simulink model "takeoffANDlandingV5_23b"  (R2023b)
settings: Solver=ode4  StartTime=0.0  StopTime=450  FixedStep=0.001  RelTol=1e-3
values from neighbouring files (symbols this model uses):
  a0 = 340.294    [basedata.m]    (also in basedata.mat; control_design.mat; landing_init.m; landing_plan.mat)
  b_ref = 2.0    (= 2)    [basedata.m]    (also in basedata.mat; control_design.mat; landing_init.m; landing_plan.mat)
  c_gear = [0.8e4, 1.4e4, 1.4e4]    [basedata.m]    (also in basedata.mat = [8000 14000 14000]; control_design.mat = [8000 14000 14000]; landing_init.m; landing_plan.mat = [8000 14000 14000])
  c_lat = [1.4e4, 2.2e4, 2.2e4]    [basedata.m]    (also in basedata.mat = [14000 22000 22000]; control_design.mat = [14000 22000 22000]; landing_init.m; landing_plan.mat = [14000 22000 22000])
  c_ref = 0.9    [basedata.m]    (also in basedata.mat; control_design.mat; landing_init.m; landing_plan.mat)
  c_roll = [0.020, 0.018, 0.018]    [basedata.m]    (also in basedata.mat = [0.02 0.018 0.018]; control_design.mat = [0.02 0.018 0.018]; landing_init.m; landing_plan.mat = [0.02 0.018 0.018])
  CD0 = 0.045    [basedata.m]    (also in basedata.mat; canshujisuan.m; control_design.mat; landing_init.m)
  CL0 = 0.083    [basedata.m]    (also in basedata.mat; control_design.mat; landing_init.m; landing_plan.mat)
  CLa = 3.80    (= 3.8)    [basedata.m]    (also in basedata.mat; canshujisuan.m = 2.5; control_design.mat; landing_init.m)
  Clb = -0.08    [basedata.m]    (also in basedata.mat; control_design.mat; landing_init.m; landing_plan.mat)
  Clda = -0.20    (= -0.2)    [basedata.m]    (also in basedata.mat; control_design.mat; landing_init.m; landing_plan.mat)
  CLde = 0.28    [basedata.m]    (also in basedata.mat; control_design.mat; landing_init.m; landing_plan.mat)
  Clp = -0.70    (= -0.7)    [basedata.m]    (also in basedata.mat; control_design.mat; landing_init.m; landing_plan.mat)
  CLq = 4.50    (= 4.5)    [basedata.m]    (also in basedata.mat; canshujisuan.m = 3; control_design.mat; landing_init.m)
  Clr = 0.08    [basedata.m]    (also in basedata.mat; control_design.mat; landing_init.m; landing_plan.mat)
  Cm0 = 0.060    (= 0.06)    [basedata.m]    (also in basedata.mat; control_design.mat; landing_init.m; landing_plan.mat)
  Cma = -0.80    (= -0.8)    [basedata.m]    (also in basedata.mat; control_design.mat; landing_init.m; landing_plan.mat)
  Cmde = -0.90    (= -0.9)    [basedata.m]    (also in basedata.mat; control_design.mat; landing_init.m; landing_plan.mat)
  Cmq = -18.0    (= -18)    [basedata.m]    (also in basedata.mat; control_design.mat; landing_init.m; landing_plan.mat)
  Cnb = 0.25    [basedata.m]    (also in basedata.mat; control_design.mat; landing_init.m; landing_plan.mat)
  Cndr = -0.15    [basedata.m]    (also in basedata.mat; control_design.mat; landing_init.m; landing_plan.mat)
  Cnp = -0.04    [basedata.m]    (also in basedata.mat; control_design.mat; landing_init.m; landing_plan.mat)
  Cnr = -0.45    [basedata.m]    (also in basedata.mat; control_design.mat; landing_init.m; landing_plan.mat)
  CSb = -0.70    (= -0.7)    [basedata.m]    (also in basedata.mat; control_design.mat; landing_init.m; landing_plan.mat)
  CSdr = 0.18    [basedata.m]    (also in basedata.mat; control_design.mat; landing_init.m; landing_plan.mat)
  CSr = 0.12    [basedata.m]    (also in basedata.mat; control_design.mat; landing_init.m; landing_plan.mat)
  D = 0.5 * rho0 * V^2 * S_ref * CD_current    [canshujisuan.m]
  D0 = 1400    [basedata.m]    (also in basedata.mat; control_design.mat = 800; landing.m; landing_init.m)
  da_max = 25    [basedata.m]    (also in basedata.mat; control_design.mat; landing_init.m; landing_plan.mat)
  da_min = -da_max    (= -25)    [basedata.m]    (also in basedata.mat; control_design.mat; landing_init.m; landing_plan.mat)
  de_max = 25    [basedata.m]    (also in basedata.mat; control_design.mat; landing_init.m; landing_plan.mat)
  de_min = -de_max    (= -25)    [basedata.m]    (also in basedata.mat; control_design.mat; landing_init.m; landing_plan.mat)
  DH = pi / 180    (= 0.0174532925199)    [basedata.m]    (also in basedata.mat; control_design.mat; landing_init.m; landing_plan.mat)
  dr_max = 25    [basedata.m]    (also in basedata.mat; control_design.mat; landing_init.m; landing_plan.mat)
  dr_min = -dr_max    (= -25)    [basedata.m]    (also in basedata.mat; control_design.mat; landing_init.m; landing_plan.mat)
  g = 9.80665    [basedata.m]    (also in basedata.mat; canshujisuan.m; control_design.mat; landing_init.m)
  ground_z = 0.0    (= 0)    [basedata.m]    (also in basedata.mat; control_design.mat; landing_init.m; landing_plan.mat)
  H_B = 132.622761894    [basedata.mat]    (also in landing_trajectory.m = H_R - R * cos(a1); landingplan.mat)
  H_C = 72.1000994005    [basedata.mat]    (also in landing_trajectory.m = H_R - R * cos(a2); landingplan.mat)
  H_climb_complete = 1000    [control_design.mat]    (also in landing.m; landing_init.m; landing_plan.mat; landingplan.mat)
  H_entry = 1000    [basedata.mat]    (also in landing_trajectory.m; landingplan.mat)
  H_exp = 20    [basedata.mat]    (also in landing_trajectory.m; landingplan.mat)
  HD = 180 / pi    (= 57.2957795131)    [basedata.m]    (also in basedata.mat; control_design.mat; landing_init.m; landing_plan.mat)
  I = [ Ixx, -Ixy, -Ixz ... (first row only)    [basedata.m]    (also in basedata.mat = [120  0  0; 0  480  0; 0  0  520]; control_design.mat = [120  0  0; 0  480  0; 0  0  520]; landing_init.m; landing_plan.mat = [120  0  0; 0  480  0; 0  0  520])
  K = 0.12    [basedata.m]    (also in basedata.mat; canshujisuan.m = 0.08; control_design.mat; landing_init.m)
  K_alpha = 7.5375    [basedata.mat]    (also in control_design.m = (((wd_pitch^2)-a24))/(2*kesi_pitch*wd_pitch); control_design.mat; controller.m = 5; landingplan.mat)
  k_gear = [1.0e5, 3.0e5, 3.0e5]    [basedata.m]    (also in basedata.mat = [100000 300000 300000]; control_design.mat = [100000 300000 300000]; landing_init.m; landing_plan.mat = [100000 300000 300000])
  Kn_pitch = -0.120095403309    [basedata.mat]    (also in control_design.m = -(2.2*g*(wd_pitch)^2)/(Tr*(((wd_pitch)^2)-a24)*V_control*a34; control_design.mat; controller.m = (2.2*wd^2*g)/(Tr*(wd^2-a24)*V_test*a34); landingplan.mat)
  Kw_pitch = -0.483749055178    [basedata.mat]    (also in control_design.m = -2*kesi_pitch*wd_pitch/a25; control_design.mat; controller.m = -(2*zeta*wd) / a25; landingplan.mat)
  m = 600.0    (= 600)    [basedata.m]    (also in basedata.mat; canshujisuan.m; control_design.mat; landing_init.m)
  mu_brake = [0.0, 0.55, 0.55]    [basedata.m]    (also in basedata.mat = [0 0.55 0.55]; control_design.mat = [0 0.55 0.55]; landing_init.m; landing_plan.mat = [0 0.55 0.55])
  phi0 = 0    [control_design.mat]    (also in landing.m; landing_init.m; landing_init.mat; landing_plan.mat)
  psi0 = 0    [control_design.mat]    (also in landing.m; landing_init.m; landing_init.mat; landing_plan.mat)
  r_left_b = r_gear_b(:,2)    [basedata.m]    (also in basedata.mat = [-0.333333333333 -0.8 0.65]; control_design.mat = [-0.333333333333 -0.8 0.65]; landing_init.m; landing_plan.mat = [-0.333333333333 -0.8 0.65])
  r_nose_b = r_gear_b(:,1)    [basedata.m]    (also in basedata.mat = [2 0 0.65]; control_design.mat = [2 0 0.65]; landing_init.m; landing_plan.mat = [2 0 0.65])
  r_right_b = r_gear_b(:,3)    [basedata.m]    (also in basedata.mat = [-0.333333333333 0.8 0.65]; control_design.mat = [-0.333333333333 0.8 0.65]; landing_init.m; landing_plan.mat = [-0.333333333333 0.8 0.65])
  rho0 = 1.225    [basedata.m]    (also in basedata.mat; canshujisuan.m; control_design.mat; landing_init.m)
  S_ref = 1.2    [basedata.m]    (also in basedata.mat; canshujisuan.m; control_design.mat; landing_init.m)
  theta0 = 0    [control_design.mat]    (also in landing.m; landing_init.m; landing_init.mat = 0.0523598775598; landing_plan.mat = 0.0523560209424)
  u0_b = 0    [control_design.mat]    (also in landing.m = 128; landing_init.m = 128; landing_init.mat = 100; landing_plan.mat = 128)
  v0_b = 0    [control_design.mat]    (also in landing.m; landing_init.m; landing_init.mat; landing_plan.mat)
  V_app = 128.516392565    [basedata.mat]    (also in landing_trajectory.m = 1.4 * Vs; landingplan.mat)
  V_cruise = 200    [basedata.m]
  v_eps = 0.20    (= 0.2)    [basedata.m]    (also in basedata.mat; control_design.mat; landing_init.m; landing_plan.mat)
  V_flare = V_shallow    [landing_trajectory.m]
  V_min = 3    [control_design.mat]    (also in landing.m; landing_init.m; landing_plan.mat; landingplan.mat)
  V_shallow = 110.156907913    [basedata.mat]    (also in landing_trajectory.m = 1.2 * Vs; landingplan.mat)
  w0_b = 0    [control_design.mat]    (also in landing.m; landing_init.m; landing_init.mat; landing_plan.mat)
  wheel_radius = 0.18    [basedata.m]    (also in basedata.mat; control_design.mat; landing_init.m; landing_plan.mat)
  WOW_on = 0.000    (= 0)    [basedata.m]    (also in basedata.mat; control_design.mat; landing_init.m; landing_plan.mat)
  Xg0 = 0    [control_design.mat]    (also in landing.m = -12000; landing_init.m = -12000; landing_init.mat = -8000; landing_plan.mat = -12000)
  Yg0 = 3    [control_design.mat]    (also in landing.m = 0; landing_init.m = 0; landing_init.mat = 0; landing_plan.mat = 0)
  Zg0 = ground_z - wheel_radius - r_gear_b(3,1) + static_deflection    [basedata.m]    (also in basedata.mat = -0.8215943; control_design.mat = -0.8215943; landing.m = -1000; landing_init.m = -1000)
undefined symbols (not defined in the file or in its folder): H_start, I_xz, I_yz, Ix_Iy, Iy_Iz, Iz_Ix, X_landing_start
libraries: simulink x54, matrix_library x19
(part 1 of 4)
settings Model: SimulationMode=accelerator  Creator=34355  LastModifiedBy=34355
settings RTWCC: GPUComputeCapability=5.0

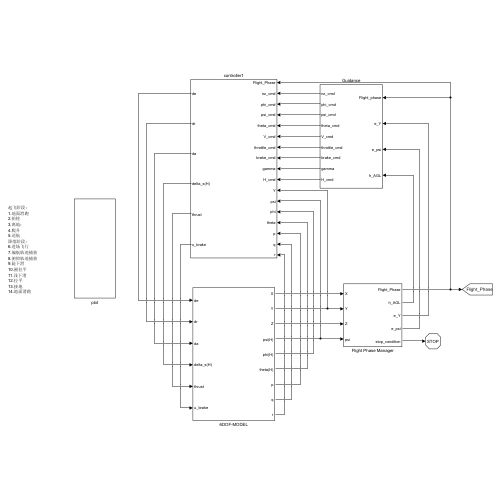
[thumbnail: Simulink's stored preview of the top-level diagram]
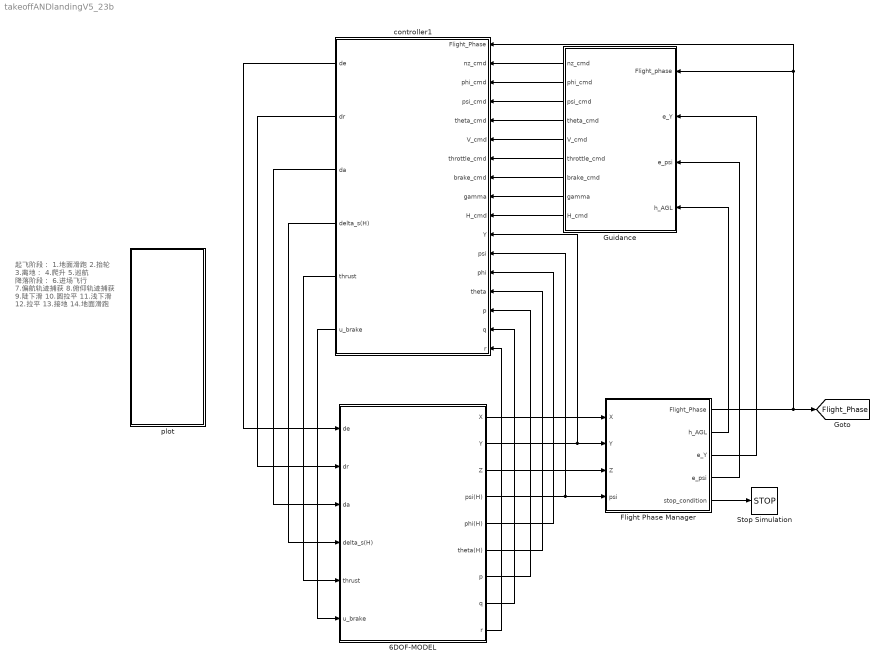
== system takeoffANDlandingV5_23b ==
  note: 起飞阶段：
      | 1.地面滑跑
      | 2.抬轮
      | 3.离地：
      | 4.爬升
      | 5.巡航
      | 降落阶段：
      | 6.进场飞行
      | 7.偏航轨迹捕获
      | 8.俯仰轨迹捕获
      | 9.陡下滑
      | 10.圆拉平
      | 11.浅下滑
      | 12.拉平
      | 13.接地
      | 14.地面滑跑
  6DOF-MODEL : Subsystem
  Flight Phase Manager : Subsystem
  Guidance : Subsystem
  Stop Simulation : Stop
  controller1 : Subsystem
  plot : Subsystem
  tag scope: Flight_Phase=global
  wires:
  controller1/1(de) -> 6DOF-MODEL/1(de)
  controller1/2(dr) -> 6DOF-MODEL/2(dr)
  controller1/3(da) -> 6DOF-MODEL/3(da)
  controller1/4(delta_s(H)) -> 6DOF-MODEL/4(delta_s(H))
  controller1/5(thrust) -> 6DOF-MODEL/5(thrust)
  controller1/6(u_brake) -> 6DOF-MODEL/6(u_brake)
  Flight Phase Manager/1(Flight_Phase) -> [Flight_Phase], Guidance/1(Flight_phase), controller1/1(Flight_Phase)
  Flight Phase Manager/3(e_Y) -> Guidance/2(e_Y)
  Flight Phase Manager/4(e_psi) -> Guidance/3(e_psi)
  Flight Phase Manager/2(h_AGL) -> Guidance/4(h_AGL)
  Guidance/1(nz_cmd) -> controller1/2(nz_cmd)
  Guidance/2(phi_cmd) -> controller1/3(phi_cmd)
  Guidance/4(theta_cmd) -> controller1/5(theta_cmd)
  Guidance/5(V_cmd) -> controller1/6(V_cmd)
  Guidance/6(throttle_cmd) -> controller1/7(throttle_cmd)
  Guidance/7(brake_cmd) -> controller1/8(brake_cmd)
  Guidance/8(gamma) -> controller1/9(gamma)
  Guidance/9(H_cmd) -> controller1/10(H_cmd)
  Flight Phase Manager/5(stop_condition) -> Stop Simulation/1
  Guidance/3(psi_cmd) -> controller1/4(psi_cmd)
  6DOF-MODEL/1(X) -> Flight Phase Manager/1(X)
  6DOF-MODEL/2(Y) -> controller1/11(Y), Flight Phase Manager/2(Y)
  6DOF-MODEL/3(Z) -> Flight Phase Manager/3(Z)
  6DOF-MODEL/4(psi(H)) -> Flight Phase Manager/4(psi), controller1/12(psi)
  6DOF-MODEL/5(phi(H)) -> controller1/13(phi)
  6DOF-MODEL/6(theta(H)) -> controller1/14(theta)
  6DOF-MODEL/7(p) -> controller1/15(p)
  6DOF-MODEL/8(q) -> controller1/16(q)
  6DOF-MODEL/9(r) -> controller1/17(r)

== system takeoffANDlandingV5_23b/6DOF-MODEL ==
  de : Inport
  dr : Inport  Port=2
  da : Inport  Port=3
  delta_s(H) : Inport  Port=4
  thrust : Inport  Port=5
  u_brake : Inport  Port=6
  AERO-PARAMETER : Subsystem
  Scope : Scope
  Scope5 : Scope
  Scope6 : Scope
  动力学 : Subsystem
  X : Outport
  Y : Outport  Port=2
  Z : Outport  Port=3
  psi(H) : Outport  Port=4
  phi(H) : Outport  Port=5
  theta(H) : Outport  Port=6
  p : Outport  Port=7
  q : Outport  Port=8
  r : Outport  Port=9
  wires:
  动力学/1(alpha(D)) -> Scope/1, AERO-PARAMETER/1(alpha(D))
  thrust/1 -> 动力学/7(thrust)
  u_brake/1 -> 动力学/9(u_brake)
  AERO-PARAMETER/1(D) -> Scope6/1, 动力学/1(D)
  AERO-PARAMETER/2(L) -> Scope5/1, 动力学/2(L)
  AERO-PARAMETER/3(S) -> 动力学/3(S)
  AERO-PARAMETER/4(MX) -> 动力学/4(MX)
  AERO-PARAMETER/5(MY) -> 动力学/5(MY)
  AERO-PARAMETER/6(MZ) -> 动力学/6(MZ)
  delta_s(H)/1 -> 动力学/8(delta_s(H))
  动力学/2(beta(D)) -> AERO-PARAMETER/2(beta(D))
  动力学/3(p) -> p/1, AERO-PARAMETER/3(p(H))
  动力学/4(q) -> q/1, AERO-PARAMETER/4(q(H))
  动力学/5(r) -> r/1, AERO-PARAMETER/5(r(H))
  de/1 -> AERO-PARAMETER/6(de(D))
  dr/1 -> AERO-PARAMETER/7(dr(D))
  da/1 -> AERO-PARAMETER/8(da)
  动力学/7(Y) -> Y/1
  动力学/8(Z) -> Z/1
  动力学/11(psi(H)) -> psi(H)/1
  动力学/10(theta(H)) -> theta(H)/1
  动力学/6(X) -> X/1
  动力学/9(phi(H)) -> phi(H)/1

== system takeoffANDlandingV5_23b/Flight Phase Manager ==
  X : Inport
  Y : Inport  Port=2
  Z : Inport  Port=3
  psi : Inport  Port=4
  Data Pre-processing : Subsystem
  Phase Logic : Stateflow chart  TreatAsAtomicUnit=on
  Flight_Phase : Outport
  h_AGL : Outport  Port=2
  e_Y : Outport  Port=3
  e_psi : Outport  Port=4
  stop_condition : Outport  Port=5
  wires:
  X/1 -> Data Pre-processing/1(X)
  Y/1 -> Data Pre-processing/2(Y)
  Z/1 -> Data Pre-processing/3(Z)
  psi/1 -> Data Pre-processing/4(psi)
  Phase Logic/1(Flight_Phase) -> Flight_Phase/1
  Data Pre-processing/1(reach_VR) -> Phase Logic/1(reach_VR)
  Data Pre-processing/2(airborne) -> Phase Logic/2(airborne)
  Data Pre-processing/3(safe_climb) -> Phase Logic/3(safe_climb)
  Data Pre-processing/4(in_cruise) -> Phase Logic/4(in_cruise)
  Data Pre-processing/5(task_mode) -> Phase Logic/5(Task_Mode)
  Data Pre-processing/6(yaw_captrue) -> Phase Logic/6(yawcapture)
  Data Pre-processing/8(in_steep) -> Phase Logic/8(in_steep)
  Data Pre-processing/9(In_round) -> Phase Logic/9(in_round)
  Data Pre-processing/10(Slight decline) -> Phase Logic/10(Slight_decline)
  Data Pre-processing/11(in_flare) -> Phase Logic/11(in_Flare)
  Data Pre-processing/12(touch_ground) -> Phase Logic/12(touch_ground)
  Data Pre-processing/13(in_ground) -> Phase Logic/13(in_ground)
  Data Pre-processing/14(h_ALG) -> h_AGL/1
  Data Pre-processing/16(e_Y) -> e_Y/1
  Data Pre-processing/15(e_psi) -> e_psi/1
  Data Pre-processing/17(stop_condition) -> stop_condition/1
  Data Pre-processing/7(pitchcaptrue) -> Phase Logic/7(pitchcaptrue)

== system takeoffANDlandingV5_23b/Guidance ==
  Flight_phase : Inport
  e_Y : Inport  Port=2
  e_psi : Inport  Port=3
  h_AGL : Inport  Port=4
  Bus Selector : BusSelector  OutputSignals=nz_cmd,phi_cmd,psi_cmd,theta_cmd,V_cmd,throttle_cmd,brake_cmd,H_cmd,gamma
  Compare To Constant : simulink/Logic and Bit Operations/Compare To Constant  relop=<=  const=5  OutDataTypeStr=boolean
  Compare To Constant1 : simulink/Logic and Bit Operations/Compare To Constant  relop=>  const=5  OutDataTypeStr=boolean
  Gain : Gain  Gain=HD
  Gain1 : Gain  Gain=HD
  Merge : Merge
  Rate Limiter : RateLimiter  RisingSlewLimit=1*DH  FallingSlewLimit=-1*DH  SampleTimeMode=inherited
  Rate Limiter1 : RateLimiter  RisingSlewLimit=10*DH  FallingSlewLimit=-10*DH  SampleTimeMode=inherited
  Rate Limiter2 : RateLimiter  RisingSlewLimit=10*DH  FallingSlewLimit=-10*DH  SampleTimeMode=inherited
  Rate Limiter3 : RateLimiter  RisingSlewLimit=0.8  FallingSlewLimit=-0.8  SampleTimeMode=inherited
  Saturation : Saturate  UpperLimit=2  LowerLimit=-2
  Saturation2 : Saturate  UpperLimit=1  LowerLimit=0
  Saturation3 : Saturate  UpperLimit=1  LowerLimit=0
  Saturation4 : Saturate  UpperLimit=250  LowerLimit=0
  Scope : Scope
  Scope8 : Scope
  Scope9 : Scope
  起飞阶段 : Subsystem
  降落阶段 : Subsystem
  nz_cmd : Outport
  phi_cmd : Outport  Port=2
  psi_cmd : Outport  Port=3
  theta_cmd : Outport  Port=4
  V_cmd : Outport  Port=5
  throttle_cmd : Outport  Port=6
  brake_cmd : Outport  Port=7
  gamma : Outport  Port=8
  H_cmd : Outport  Port=9
  wires:
  Bus Selector/5 -> Saturation4/1  "<V_cmd>"
  Bus Selector/4 -> Rate Limiter/1  "<theta_cmd>"
  Saturation4/1 -> V_cmd/1
  Bus Selector/7 -> Saturation3/1  "<brake_cmd>"
  Rate Limiter2/1 -> psi_cmd/1
  Saturation/1 -> Rate Limiter3/1
  Saturation3/1 -> brake_cmd/1
  Saturation2/1 -> throttle_cmd/1
  Merge/1 -> Bus Selector/1
  [vzg] -> 起飞阶段/8(vzg), 降落阶段/6(vzg)
  Rate Limiter/1 -> theta_cmd/1, Gain1/1
  Bus Selector/2 -> Rate Limiter1/1  "<phi_cmd>"
  Bus Selector/8 -> H_cmd/1, Scope9/1  "<H_cmd>"
  [theta_eular] -> 降落阶段/8(theta_eular), 起飞阶段/10(theta_eular)
  降落阶段/1(Cmd_Bus) -> Merge/2
  Bus Selector/1 -> Saturation/1  "<nz_cmd>"
  h_AGL/1 -> 起飞阶段/7(h_ALG), 降落阶段/2(h_AGL)
  [vxg] -> 降落阶段/9(Vg)
  [phi_eular] -> 起飞阶段/9(phi_eular), 降落阶段/7(phi_eular)
  起飞阶段/1(Cmd_Bus) -> Merge/1
  Flight_phase/1 -> Compare To Constant/1, 起飞阶段/1(Flight_phase), 降落阶段/1(Flight_phase), Compare To Constant1/1
  Compare To Constant/1 -> 起飞阶段/Enable
  [r] -> 起飞阶段/4(r)
  [Vwind_ground] -> 起飞阶段/5(Vwind_ground), 降落阶段/3(Vwind_ground)
  e_psi/1 -> 起飞阶段/3(e_psi)
  Gain/1 -> Scope8/1
  e_Y/1 -> 起飞阶段/2(e_Y)
  Bus Selector/9 -> gamma/1, Gain/1  "<gamma>"
  Compare To Constant1/1 -> 降落阶段/Enable
  [Va_safe] -> 起飞阶段/6(Va_safe), 降落阶段/4(Va_safe)
  Rate Limiter3/1 -> nz_cmd/1
  Bus Selector/6 -> Saturation2/1  "<throttle_cmd>"
  Rate Limiter1/1 -> phi_cmd/1
  [X_positon] -> 降落阶段/5(x_pos)
  Bus Selector/3 -> Rate Limiter2/1  "<psi_cmd>"
  Gain1/1 -> Scope/1

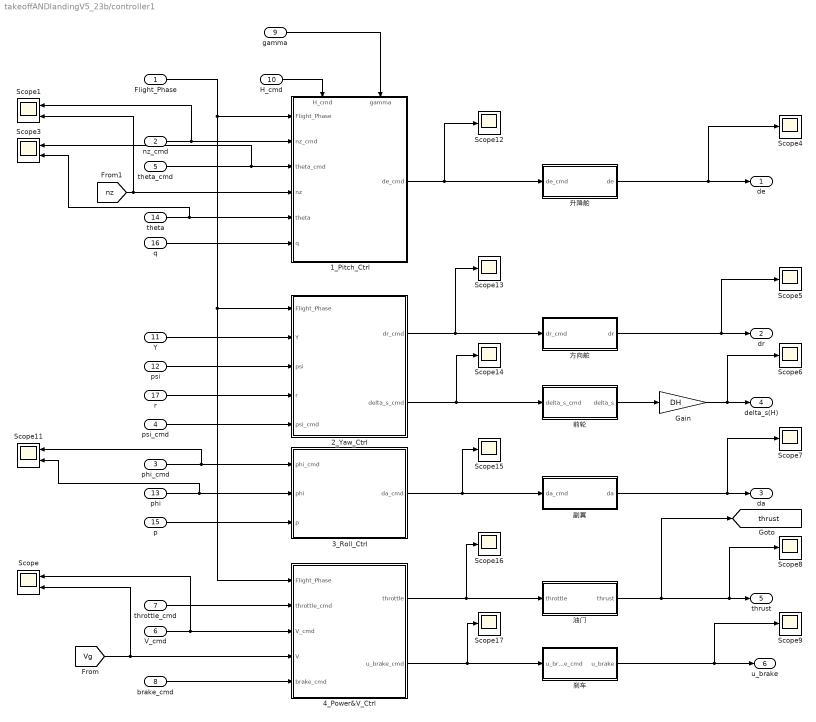
== system takeoffANDlandingV5_23b/controller1 ==
  Flight_Phase : Inport
  nz_cmd : Inport  Port=2
  phi_cmd : Inport  Port=3
  psi_cmd : Inport  Port=4
  theta_cmd : Inport  Port=5
  V_cmd : Inport  Port=6
  throttle_cmd : Inport  Port=7
  brake_cmd : Inport  Port=8
  gamma : Inport  Port=9
  H_cmd : Inport  Port=10
  Y : Inport  Port=11
  psi : Inport  Port=12
  phi : Inport  Port=13
  theta : Inport  Port=14
  p : Inport  Port=15
  q : Inport  Port=16
  r : Inport  Port=17
  1_Pitch_Ctrl : Subsystem
      settings: PortSchema="{\"entries\":[{\"content\":{\"sides\":[{\"content\":{\"connectorIds\":[\"In1\",\"In2\",\"In3\",\"In4\",\"In5\",\"In6\"]},\"type\":\"ConnectorPlacement.EquallySpacedRectSide\",\"uuid\":\"27d13232-9f89-4ac1-9c77-5758657de7c7\"},{\"content\":{\"connectorIds\":[\"Out1\"],\"side\":\"RIGHT\"},\"type\":\"ConnectorPlacement.EquallySpacedRectSide\",\"uuid\":\"ae62ad8c-a405-4422-b5ec-9ac723f70591\"},{\"content\":{\"connectorIds\":[\"In7\",\"In8\"],\"side\":\"TOP\"},\"type\":\"ConnectorPlacement.EquallySpacedRectSide\",\"uuid\":\"4cebe0f4-d768-4fb6-931c-2fd4183255b7\"}]},\"type\":\"ConnectorPlacement.EquallySpacedConnector\",\"uuid\":\"2c44e0df-7f94-4dab-9232-216c905b911f\"}],\"packageUris\":[\"http://schema.mathworks.com/mf0/Connector/R2020b\"],\"version\":\"1.0\"}"
  2_Yaw_Ctrl : Subsystem
  3_Roll_Ctrl : Subsystem
  4_Power&V_Ctrl : Subsystem
  Gain : Gain  Gain=DH
  Scope{,1,3,11} (4 alike) : Scope  NumInputPorts=2
  Scope{4..9,12..17} (12 alike) : Scope
  刹车 : Subsystem
  前轮 : Subsystem
  副翼 : Subsystem
  升降舵 : Subsystem
  方向舵 : Subsystem
  油门 : Subsystem
  de : Outport
  dr : Outport  Port=2
  da : Outport  Port=3
  delta_s(H) : Outport  Port=4
  thrust : Outport  Port=5
  u_brake : Outport  Port=6
  tag scope: thrust=global
  wires:
  phi_cmd/1 -> Scope11/1, 3_Roll_Ctrl/1(phi_cmd)
  phi/1 -> Scope11/2, 3_Roll_Ctrl/2(phi)
  p/1 -> 3_Roll_Ctrl/3(p)
  brake_cmd/1 -> 4_Power&V_Ctrl/5(brake_cmd)
  4_Power&V_Ctrl/1(throttle) -> 油门/1(throttle), Scope16/1
  Flight_Phase/1 -> 1_Pitch_Ctrl/1(Flight_Phase), 4_Power&V_Ctrl/1(Flight_Phase), 2_Yaw_Ctrl/1(Flight_Phase)
  nz_cmd/1 -> Scope1/1, 1_Pitch_Ctrl/2(nz_cmd)
  [nz] -> Scope1/2, 1_Pitch_Ctrl/4(nz)
  q/1 -> 1_Pitch_Ctrl/6(q)
  V_cmd/1 -> 4_Power&V_Ctrl/3(V_cmd), Scope/1
  [Vg] -> Scope/2, 4_Power&V_Ctrl/4(V)
  Gain/1 -> Scope6/1, delta_s(H)/1
  theta_cmd/1 -> Scope3/1, 1_Pitch_Ctrl/3(theta_cmd)
  1_Pitch_Ctrl/1(de_cmd) -> 升降舵/1(de_cmd), Scope12/1
  2_Yaw_Ctrl/1(dr_cmd) -> Scope13/1, 方向舵/1(dr_cmd)
  2_Yaw_Ctrl/2(delta_s_cmd) -> Scope14/1, 前轮/1(delta_s_cmd)
  3_Roll_Ctrl/1(da_cmd) -> Scope15/1, 副翼/1(da_cmd)
  4_Power&V_Ctrl/2(u_brake_cmd) -> 刹车/1(u_brake_cmd), Scope17/1
  theta/1 -> Scope3/2, 1_Pitch_Ctrl/5(theta)
  throttle_cmd/1 -> 4_Power&V_Ctrl/2(throttle_cmd)
  Y/1 -> 2_Yaw_Ctrl/2(Y)
  psi/1 -> 2_Yaw_Ctrl/3(psi)
  r/1 -> 2_Yaw_Ctrl/4(r)
  升降舵/1(de) -> Scope4/1, de/1
  方向舵/1(dr) -> Scope5/1, dr/1
  前轮/1(delta_s) -> Gain/1
  副翼/1(da) -> Scope7/1, da/1
  油门/1(thrust) -> [thrust], Scope8/1, thrust/1
  刹车/1(u_brake) -> Scope9/1, u_brake/1
  H_cmd/1 -> 1_Pitch_Ctrl/7(H_cmd)
  gamma/1 -> 1_Pitch_Ctrl/8(gamma)
  psi_cmd/1 -> 2_Yaw_Ctrl/5(psi_cmd)

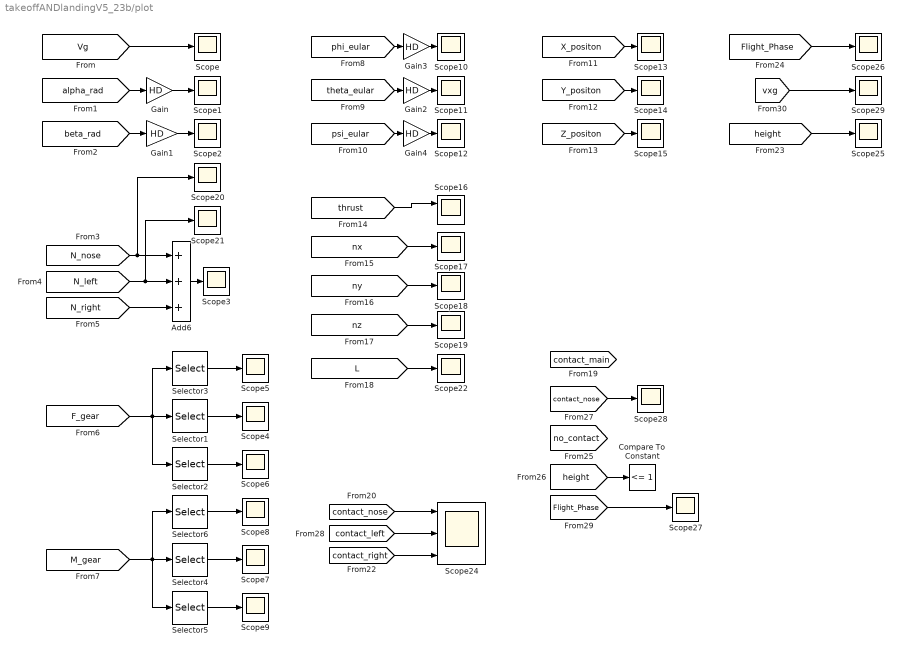
== system takeoffANDlandingV5_23b/plot ==
  Add6 : Sum  Inputs=+++
  Compare To Constant : simulink/Logic and Bit Operations/Compare To Constant  relop=<=  const=1  OutDataTypeStr=boolean
  Gain{,1..4} (5 alike) : Gain  Gain=HD
  Scope{,1..15,17..22,25..29} (27 alike) : Scope
  Scope16 : Scope  NumInputPorts=2
  Scope24 : Scope  NumInputPorts=3
  Selector1 : Selector  InputPortWidth=3  IndexOptions=Index vector (dialog)  Indices=2  OutputSizes=1
  Selector2 : Selector  InputPortWidth=3  IndexOptions=Index vector (dialog)  Indices=3  OutputSizes=1
  Selector3 : Selector  InputPortWidth=3  IndexOptions=Index vector (dialog)  Indices=1  OutputSizes=1
  Selector4 : Selector  InputPortWidth=3  IndexOptions=Index vector (dialog)  Indices=2  OutputSizes=1
  Selector5 : Selector  InputPortWidth=3  IndexOptions=Index vector (dialog)  Indices=3  OutputSizes=1
  Selector6 : Selector  InputPortWidth=3  IndexOptions=Index vector (dialog)  Indices=1  OutputSizes=1
  wires:
  [N_nose] -> Add6/1, Scope20/1
  [N_left] -> Scope21/1, Add6/2
  [N_right] -> Add6/3
  [Vg] -> Scope/1
  [alpha_rad] -> Gain/1
  [beta_rad] -> Gain1/1
  Add6/1 -> Scope3/1
  Selector3/1 -> Scope5/1
  Selector2/1 -> Scope6/1
  Selector1/1 -> Scope4/1
  [F_gear] -> Selector2/1, Selector1/1, Selector3/1
  Selector6/1 -> Scope8/1
  Selector4/1 -> Scope7/1
  [M_gear] -> Selector6/1, Selector4/1, Selector5/1
  Selector5/1 -> Scope9/1
  [psi_eular] -> Gain4/1
  [theta_eular] -> Gain2/1
  [phi_eular] -> Gain3/1
  Gain1/1 -> Scope2/1
  Gain/1 -> Scope1/1
  Gain2/1 -> Scope11/1
  [Y_positon] -> Scope14/1
  [X_positon] -> Scope13/1
  [Z_positon] -> Scope15/1
  Gain3/1 -> Scope10/1
  Gain4/1 -> Scope12/1
  [thrust] -> Scope16/1
  [nx] -> Scope17/1
  [ny] -> Scope18/1
  [nz] -> Scope19/1
  [L] -> Scope22/1
  [height] -> Scope25/1
  [height] -> Compare To Constant/1
  [contact_left] -> Scope24/2
  [contact_right] -> Scope24/3
  [Flight_Phase] -> Scope26/1
  [contact_nose] -> Scope28/1
  [contact_nose] -> Scope24/1
  [Flight_Phase] -> Scope27/1
  [vxg] -> Scope29/1

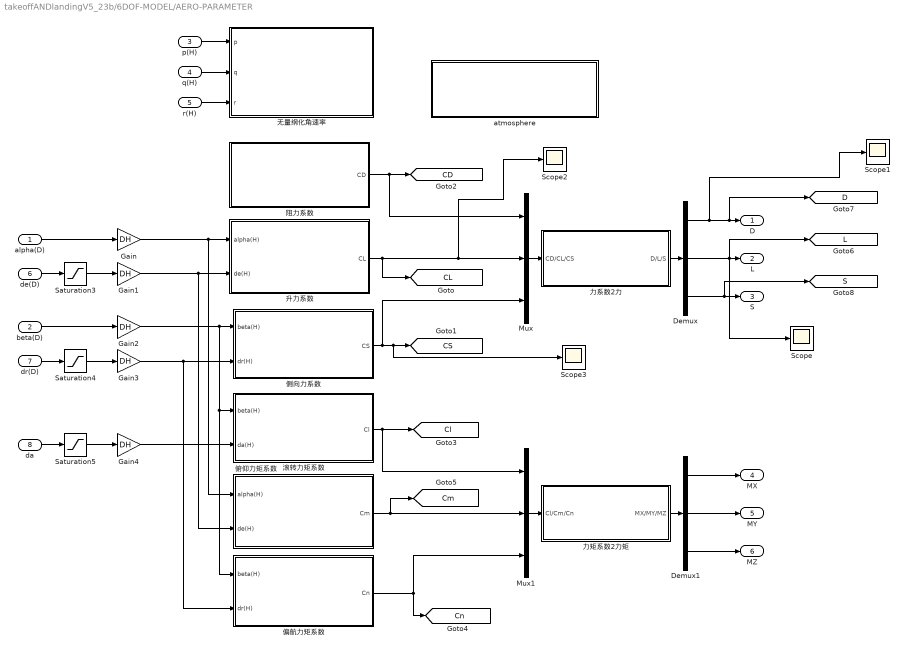
== system takeoffANDlandingV5_23b/6DOF-MODEL/AERO-PARAMETER ==
  alpha(D) : Inport
  beta(D) : Inport  Port=2
  p(H) : Inport  Port=3
  q(H) : Inport  Port=4
  r(H) : Inport  Port=5
  de(D) : Inport  Port=6
  dr(D) : Inport  Port=7
  da : Inport  Port=8
  Demux : Demux  Outputs=3
  Demux1 : Demux  Outputs=3
  Gain{,1..4} (5 alike) : Gain  Gain=DH
  Mux : Mux  Inputs=3
  Mux1 : Mux  Inputs=3
  Saturation3 : Saturate  UpperLimit=de_max  LowerLimit=de_min
  Saturation4 : Saturate  UpperLimit=dr_max  LowerLimit=dr_min
  Saturation5 : Saturate  UpperLimit=da_max  LowerLimit=da_min
  Scope{,1..3} (4 alike) : Scope
  atmosphere : Subsystem
  侧向力系数 : Subsystem
  俯仰力矩系数 : Subsystem
  偏航力矩系数 : Subsystem
  力矩系数2力矩 : Subsystem
  力系数2力 : Subsystem
  升力系数 : Subsystem
  无量纲化角速率 : Subsystem
  滚转力矩系数 : Subsystem
  阻力系数 : Subsystem
  D : Outport
  L : Outport  Port=2
  S : Outport  Port=3
  MX : Outport  Port=4
  MY : Outport  Port=5
  MZ : Outport  Port=6
  tag scope: CD=global, CL=global, CS=global, Cl=global, Cm=global, Cn=global, D=global, L=global, S=global
  wires:
  升力系数/1(CL) -> [CL], Scope2/1, Mux/2
  侧向力系数/1(CS) -> Mux/3, Scope3/1, [CS]
  da/1 -> Saturation5/1
  Saturation5/1 -> Gain4/1
  Saturation4/1 -> Gain3/1
  dr(D)/1 -> Saturation4/1
  de(D)/1 -> Saturation3/1
  Saturation3/1 -> Gain1/1
  beta(D)/1 -> Gain2/1
  alpha(D)/1 -> Gain/1
  Gain/1 -> 升力系数/1(alpha(H)), 俯仰力矩系数/1(alpha(H))
  Gain1/1 -> 升力系数/2(de(H)), 俯仰力矩系数/2(de(H))
  Gain2/1 -> 侧向力系数/1(beta(H)), 偏航力矩系数/1(beta(H)), 滚转力矩系数/1(beta(H))
  Gain3/1 -> 侧向力系数/2(dr(H)), 偏航力矩系数/2(dr(H))
  Gain4/1 -> 滚转力矩系数/2(da(H))
  p(H)/1 -> 无量纲化角速率/1(p)
  q(H)/1 -> 无量纲化角速率/2(q)
  r(H)/1 -> 无量纲化角速率/3(r)
  阻力系数/1(CD) -> Mux/1, [CD]
  滚转力矩系数/1(Cl) -> [Cl], Mux1/1
  俯仰力矩系数/1(Cm) -> Mux1/2, [Cm]
  偏航力矩系数/1(Cn) -> [Cn], Mux1/3
  Mux/1 -> 力系数2力/1(CD/CL/CS)
  Mux1/1 -> 力矩系数2力矩/1(Cl/Cm/Cn)
  Demux/2 -> Scope/1, [L], L/1
  力系数2力/1(D/L/S) -> Demux/1
  Demux/1 -> Scope1/1, [D], D/1
  Demux/3 -> [S], S/1
  力矩系数2力矩/1(MX/MY/MZ) -> Demux1/1
  Demux1/1 -> MX/1
  Demux1/2 -> MY/1
  Demux1/3 -> MZ/1

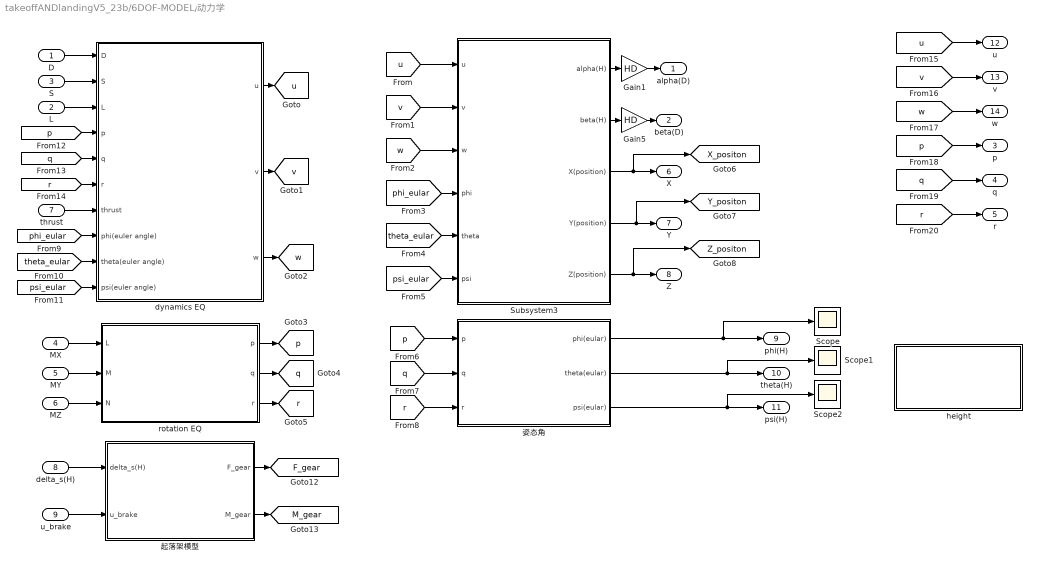
== system takeoffANDlandingV5_23b/6DOF-MODEL/动力学 ==
  D : Inport
  L : Inport  Port=2
  S : Inport  Port=3
  MX : Inport  Port=4
  MY : Inport  Port=5
  MZ : Inport  Port=6
  thrust : Inport  Port=7
  delta_s(H) : Inport  Port=8
  u_brake : Inport  Port=9
  Gain1 : Gain  Gain=HD
  Gain5 : Gain  Gain=HD
  Scope : Scope
  Scope1 : Scope
  Scope2 : Scope
  Subsystem3 : Subsystem
  dynamics EQ : Subsystem
  height : Subsystem
  rotation EQ : Subsystem
  姿态角 : Subsystem
  起落架模型 : Subsystem
  alpha(D) : Outport
  beta(D) : Outport  Port=2
  p : Outport  Port=3
  q : Outport  Port=4
  r : Outport  Port=5
  X : Outport  Port=6
  Y : Outport  Port=7
  Z : Outport  Port=8
  phi(H) : Outport  Port=9
  theta(H) : Outport  Port=10
  psi(H) : Outport  Port=11
  u : Outport  Port=12
  v : Outport  Port=13
  w : Outport  Port=14
  tag scope: F_gear=global, M_gear=global, X_positon=global, Y_positon=global, Z_positon=global, p=global, q=global, r=global, u=global, v=global, w=global
  wires:
  姿态角/1(phi(eular)) -> Scope/1, phi(H)/1
  姿态角/2(theta(eular)) -> theta(H)/1, Scope1/1
  姿态角/3(psi(eular)) -> psi(H)/1, Scope2/1
  Gain5/1 -> beta(D)/1
  Gain1/1 -> alpha(D)/1
  [u] -> u/1
  [v] -> v/1
  [w] -> w/1
  [p] -> p/1
  [q] -> q/1
  [r] -> r/1
  起落架模型/1(F_gear) -> [F_gear]
  起落架模型/2(M_gear) -> [M_gear]
  MX/1 -> rotation EQ/1(L)
  MY/1 -> rotation EQ/2(M)
  MZ/1 -> rotation EQ/3(N)
  D/1 -> dynamics EQ/1(D)
  S/1 -> dynamics EQ/2(S)
  L/1 -> dynamics EQ/3(L)
  [p] -> dynamics EQ/4(p)
  [q] -> dynamics EQ/5(q)
  [r] -> dynamics EQ/6(r)
  thrust/1 -> dynamics EQ/7(thrust)
  [phi_eular] -> dynamics EQ/8(phi(euler angle))
  [theta_eular] -> dynamics EQ/9(theta(euler angle))
  [psi_eular] -> dynamics EQ/10(psi(euler angle))
  dynamics EQ/1(u) -> [u]
  dynamics EQ/2(v) -> [v]
  dynamics EQ/3(w) -> [w]
  [u] -> Subsystem3/1(u)
  [v] -> Subsystem3/2(v)
  [w] -> Subsystem3/3(w)
  [phi_eular] -> Subsystem3/4(phi)
  [theta_eular] -> Subsystem3/5(theta)
  [psi_eular] -> Subsystem3/6(psi)
  Subsystem3/1(alpha(H)) -> Gain1/1
  Subsystem3/2(beta(H)) -> Gain5/1
  Subsystem3/3(X(position)) -> [X_positon], X/1
  Subsystem3/4(Y(position)) -> [Y_positon], Y/1
  Subsystem3/5(Z(position)) -> [Z_positon], Z/1
  delta_s(H)/1 -> 起落架模型/1(delta_s(H))
  u_brake/1 -> 起落架模型/2(u_brake)
  rotation EQ/1(p) -> [p]
  rotation EQ/2(q) -> [q]
  rotation EQ/3(r) -> [r]
  [p] -> 姿态角/1(p)
  [q] -> 姿态角/2(q)
  [r] -> 姿态角/3(r)

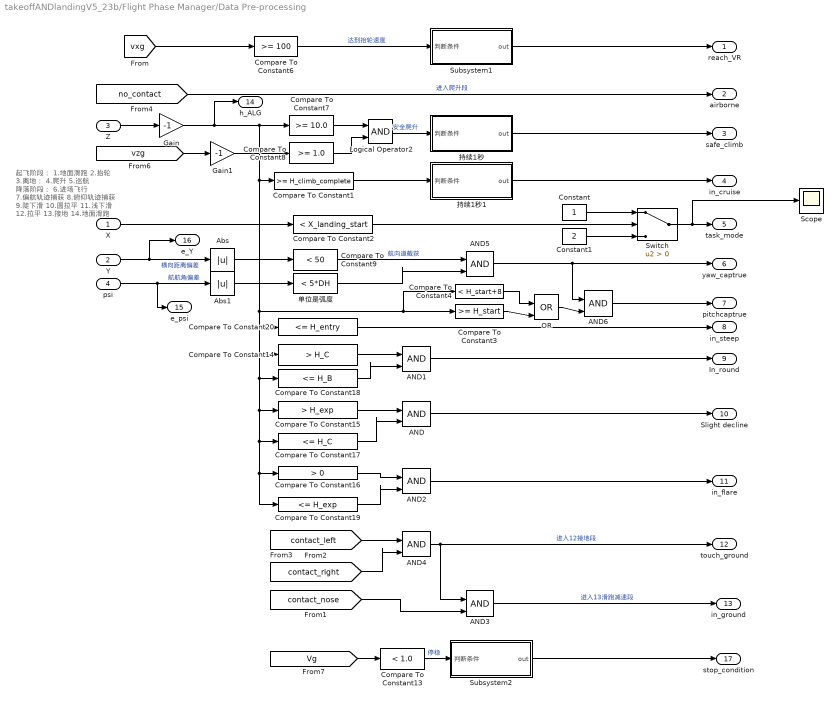
== system takeoffANDlandingV5_23b/Flight Phase Manager/Data Pre-processing ==
  note: 起飞阶段：
      | 1.地面滑跑
      | 2.抬轮
      | 3.离地：
      | 4.爬升
      | 5.巡航
      | 降落阶段：
      | 6.进场飞行
      | 7.偏航轨迹捕获
      | 8.俯仰轨迹捕获
      | 9.陡下滑
      | 10.圆拉平
      | 11.浅下滑
      | 12.拉平
      | 13.接地
      | 14.地面滑跑
  X : Inport
  Y : Inport  Port=2
  Z : Inport  Port=3
  psi : Inport  Port=4
  AND{,1..6} (7 alike) : Logic  IconShape=distinctive  AllPortsSameDT=off  OutDataTypeStr=boolean
  Abs : Abs  SaturateOnIntegerOverflow=off
  Abs1 : Abs  SaturateOnIntegerOverflow=off
  Compare To Constant1 : simulink/Logic and Bit Operations/Compare To Constant  relop=>=  const=H_climb_complete  OutDataTypeStr=boolean
  Compare To Constant13 : simulink/Logic and Bit Operations/Compare To Constant  relop=<  const=1.0  OutDataTypeStr=boolean
  Compare To Constant14 : simulink/Logic and Bit Operations/Compare To Constant  relop=>  const=H_C  OutDataTypeStr=boolean
  Compare To Constant15 : simulink/Logic and Bit Operations/Compare To Constant  relop=>  const=H_exp  OutDataTypeStr=boolean
  Compare To Constant16 : simulink/Logic and Bit Operations/Compare To Constant  relop=>  const=0  OutDataTypeStr=boolean
  Compare To Constant17 : simulink/Logic and Bit Operations/Compare To Constant  relop=<=  const=H_C  OutDataTypeStr=boolean
  Compare To Constant18 : simulink/Logic and Bit Operations/Compare To Constant  relop=<=  const=H_B  OutDataTypeStr=boolean
  Compare To Constant19 : simulink/Logic and Bit Operations/Compare To Constant  relop=<=  const=H_exp  OutDataTypeStr=boolean
  Compare To Constant2 : simulink/Logic and Bit Operations/Compare To Constant  relop=<  const=X_landing_start  OutDataTypeStr=boolean
  Compare To Constant20 : simulink/Logic and Bit Operations/Compare To Constant  relop=<=  const=H_entry  OutDataTypeStr=boolean
  Compare To Constant3 : simulink/Logic and Bit Operations/Compare To Constant  relop=>=  const=H_start  OutDataTypeStr=boolean
  Compare To Constant4 : simulink/Logic and Bit Operations/Compare To Constant  relop=<  const=H_start+8  OutDataTypeStr=boolean
  Compare To Constant6 : simulink/Logic and Bit Operations/Compare To Constant  relop=>=  const=100  OutDataTypeStr=boolean
  Compare To Constant7 : simulink/Logic and Bit Operations/Compare To Constant  relop=>=  const=10.0  OutDataTypeStr=boolean
  Compare To Constant8 : simulink/Logic and Bit Operations/Compare To Constant  relop=>=  const=1.0  OutDataTypeStr=boolean
  Compare To Constant9 : simulink/Logic and Bit Operations/Compare To Constant  relop=<  const=50  OutDataTypeStr=boolean
  Constant : Constant
  Constant1 : Constant  Value=2
  Gain : Gain  Gain=-1
  Gain1 : Gain  Gain=-1
  Logical Operator2 : Logic  AllPortsSameDT=off  OutDataTypeStr=boolean
  OR : Logic  Operator=OR  IconShape=distinctive  AllPortsSameDT=off  OutDataTypeStr=boolean
  Scope : Scope
  Subsystem1 : Subsystem
  Subsystem2 : Subsystem
  Switch : Switch  Criteria=u2 > Threshold  SaturateOnIntegerOverflow=off  InputSameDT=off
  单位是弧度 : simulink/Logic and Bit Operations/Compare To Constant  relop=<  const=5*DH  OutDataTypeStr=boolean
  持续1秒 : Subsystem
  持续1秒1 : Subsystem
  reach_VR : Outport
  airborne : Outport  Port=2
  safe_climb : Outport  Port=3
  in_cruise : Outport  Port=4
  task_mode : Outport  Port=5
  yaw_captrue : Outport  Port=6
  pitchcaptrue : Outport  Port=7
  in_steep : Outport  Port=8
  In_round : Outport  Port=9
  Slight decline : Outport  Port=10
  in_flare : Outport  Port=11
  touch_ground : Outport  Port=12
  in_ground : Outport  Port=13
  h_ALG : Outport  Port=14
  e_psi : Outport  Port=15
  e_Y : Outport  Port=16
  stop_condition : Outport  Port=17
  wires:
  Compare To Constant8/1 -> Logical Operator2/2
  Compare To Constant7/1 -> Logical Operator2/1
  持续1秒/1(out) -> safe_climb/1
  Logical Operator2/1 -> 持续1秒/1(判断条件)  "安全爬升"
  Subsystem1/1(out) -> reach_VR/1
  Compare To Constant6/1 -> Subsystem1/1(判断条件)  "达到抬轮速度"
  Compare To Constant15/1 -> AND/1
  AND/1 -> Slight decline/1
  Compare To Constant17/1 -> AND/2
  AND1/1 -> In_round/1
  Compare To Constant14/1 -> AND1/1
  Compare To Constant18/1 -> AND1/2
  Compare To Constant16/1 -> AND2/1
  AND2/1 -> in_flare/1
  Compare To Constant19/1 -> AND2/2
  X/1 -> Compare To Constant2/1
  Compare To Constant20/1 -> in_steep/1
  [contact_right] -> AND4/2
  [contact_left] -> AND4/1
  AND3/1 -> in_ground/1  "进入13滑跑减速段"
  AND4/1 -> AND3/1, touch_ground/1  "进入12接地段"
  [no_contact] -> airborne/1  "进入爬升段"
  [vxg] -> Compare To Constant6/1
  [vzg] -> Gain1/1
  Gain/1 -> h_ALG/1, Compare To Constant7/1, Compare To Constant1/1, Compare To Constant4/1, Compare To Constant3/1, Compare To Constant19/1, Compare To Constant16/1, Compare To Constant17/1, Compare To Constant15/1, Compare To Constant18/1, Compare To Constant14/1, Compare To Constant20/1
  Compare To Constant1/1 -> 持续1秒1/1(判断条件)
  持续1秒1/1(out) -> in_cruise/1
  Z/1 -> Gain/1
  [contact_nose] -> AND3/2
  psi/1 -> e_psi/1, Abs1/1  "航航角偏差"
  Y/1 -> e_Y/1, Abs/1  "横向距离偏差"
  Abs/1 -> Compare To Constant9/1
  Abs1/1 -> 单位是弧度/1
  Switch/1 -> Scope/1, task_mode/1
  Constant/1 -> Switch/1
  Constant1/1 -> Switch/3
  Gain1/1 -> Compare To Constant8/1
  [Vg] -> Compare To Constant13/1
  Compare To Constant13/1 -> Subsystem2/1(判断条件)  "停稳"
  Subsystem2/1(out) -> stop_condition/1
  Compare To Constant2/1 -> Switch/2
  Compare To Constant9/1 -> AND5/1  "航向道截获"
  单位是弧度/1 -> AND5/2
  AND5/1 -> AND6/1, yaw_captrue/1
  AND6/1 -> pitchcaptrue/1
  Compare To Constant3/1 -> OR/2
  OR/1 -> AND6/2
  Compare To Constant4/1 -> OR/1

== system takeoffANDlandingV5_23b/Guidance/起飞阶段 ==
  Flight_phase : Inport
  e_Y : Inport  Port=2
  e_psi : Inport  Port=3
  r : Inport  Port=4
  Vwind_ground : Inport  Port=5
  Va_safe : Inport  Port=6
  h_ALG : Inport  Port=7
  vzg : Inport  Port=8
  phi_eular : Inport  Port=9
  theta_eular : Inport  Port=10
  Enable : EnablePort
  AND : Logic  IconShape=distinctive  AllPortsSameDT=off  OutDataTypeStr=boolean
  Compare To Constant : simulink/Logic and Bit Operations/Compare To Constant  relop===  const=1  OutDataTypeStr=boolean
  Compare To Constant1 : simulink/Logic and Bit Operations/Compare To Constant  relop=>=  const=2  OutDataTypeStr=boolean
  Compare To Constant2 : simulink/Logic and Bit Operations/Compare To Constant  relop=<=  const=4  OutDataTypeStr=boolean
  Compare To Constant3 : simulink/Logic and Bit Operations/Compare To Constant  relop===  const=5  OutDataTypeStr=boolean
  Merge : Merge  Inputs=3
  地面滑跑阶段(1) : Subsystem
  巡航阶段(5) : Subsystem  TreatAsAtomicUnit=on
  抬轮离地爬升阶段(2/3/4) : Subsystem  TreatAsAtomicUnit=on
  Cmd_Bus : Outport
  wires:
  抬轮离地爬升阶段(2/3/4)/1(Cmd_Bus) -> Merge/2
  地面滑跑阶段(1)/1(Cmd_Bus) -> Merge/1
  Merge/1 -> Cmd_Bus/1
  巡航阶段(5)/1(Cmd_Bus) -> Merge/3
  Flight_phase/1 -> Compare To Constant3/1, Compare To Constant2/1, Compare To Constant1/1, Compare To Constant/1
  Compare To Constant/1 -> 地面滑跑阶段(1)/Enable
  Compare To Constant1/1 -> AND/1
  Compare To Constant2/1 -> AND/2
  AND/1 -> 抬轮离地爬升阶段(2/3/4)/Enable
  Compare To Constant3/1 -> 巡航阶段(5)/Enable
  e_Y/1 -> 地面滑跑阶段(1)/1(e_Y)
  e_psi/1 -> 地面滑跑阶段(1)/2(e_psi)
  r/1 -> 地面滑跑阶段(1)/3(r)
  Vwind_ground/1 -> 抬轮离地爬升阶段(2/3/4)/1(Vwind_ground), 巡航阶段(5)/1(Vwind_ground)
  Va_safe/1 -> 巡航阶段(5)/2(Va_safe), 抬轮离地爬升阶段(2/3/4)/2(Va_safe)
  h_ALG/1 -> 巡航阶段(5)/3(h_ALG)
  vzg/1 -> 巡航阶段(5)/4(vzg)
  phi_eular/1 -> 巡航阶段(5)/5(phi_eular)
  theta_eular/1 -> 巡航阶段(5)/6(theta_eular)

== system takeoffANDlandingV5_23b/Guidance/降落阶段 ==
  note: 起飞阶段：
      | 1.地面滑跑
      | 2.抬轮
      | 3.离地：
      | 4.爬升
      | 5.巡航
      | 降落阶段：
      | 6.进场飞行
      | 7.偏航轨迹捕获
      | 8.俯仰轨迹捕获
      | 9.陡下滑
      | 10.圆拉平
      | 11.浅下滑
      | 12.拉平
      | 13.接地
      | 14.地面滑跑
  Flight_phase : Inport
  h_AGL : Inport  Port=2
  Vwind_ground : Inport  Port=3
  Va_safe : Inport  Port=4
  x_pos : Inport  Port=5
  vzg : Inport  Port=6
  phi_eular : Inport  Port=7
  theta_eular : Inport  Port=8
  Vg : Inport  Port=9
  Enable : EnablePort
  AND : Logic  IconShape=distinctive  AllPortsSameDT=off  OutDataTypeStr=boolean
  Compare To Constant : simulink/Logic and Bit Operations/Compare To Constant  relop=<=  const=8  OutDataTypeStr=boolean
  Compare To Constant1 : simulink/Logic and Bit Operations/Compare To Constant  relop=<=  const=11  OutDataTypeStr=boolean
  Compare To Constant2 : simulink/Logic and Bit Operations/Compare To Constant  relop=>  const=8  OutDataTypeStr=boolean
  Compare To Constant3 : simulink/Logic and Bit Operations/Compare To Constant  relop=>  const=11  OutDataTypeStr=boolean
  MATLAB Function : MATLAB Function  TreatAsAtomicUnit=on
  Merge : Merge  Inputs=3
  拉平/接地/滑跑刹车阶段(12/13/14) : Subsystem  TreatAsAtomicUnit=on
  进场/轨迹捕获阶段(6/7/8) : Subsystem  TreatAsAtomicUnit=on
  陡下滑/圆拉平/浅下滑阶段(8/9/10) : Subsystem  TreatAsAtomicUnit=on
  Cmd_Bus : Outport
  wires:
  陡下滑/圆拉平/浅下滑阶段(8/9/10)/1(Cmd_Bus) -> Merge/2
  x_pos/1 -> MATLAB Function/2(X)
  MATLAB Function/2(H_cmd) -> 进场/轨迹捕获阶段(6/7/8)/8(H_cmd), 陡下滑/圆拉平/浅下滑阶段(8/9/10)/9(H_cmd), 拉平/接地/滑跑刹车阶段(12/13/14)/3(H_cmd)
  Flight_phase/1 -> Compare To Constant1/1, Compare To Constant2/1, 拉平/接地/滑跑刹车阶段(12/13/14)/1(Flight_Phase), Compare To Constant3/1, 陡下滑/圆拉平/浅下滑阶段(8/9/10)/3(Flight_phase), Compare To Constant/1, MATLAB Function/1(Flight_Phase)
  Merge/1 -> Cmd_Bus/1
  Compare To Constant2/1 -> AND/2
  vzg/1 -> 进场/轨迹捕获阶段(6/7/8)/4(vzg), 陡下滑/圆拉平/浅下滑阶段(8/9/10)/5(vzg)
  AND/1 -> 陡下滑/圆拉平/浅下滑阶段(8/9/10)/Enable
  h_AGL/1 -> 进场/轨迹捕获阶段(6/7/8)/3(h_ALG), 陡下滑/圆拉平/浅下滑阶段(8/9/10)/4(h_ALG), MATLAB Function/3(h_AGL)
  theta_eular/1 -> 陡下滑/圆拉平/浅下滑阶段(8/9/10)/7(theta_eular), 进场/轨迹捕获阶段(6/7/8)/6(theta_eular)
  Vwind_ground/1 -> 进场/轨迹捕获阶段(6/7/8)/1(Vwind_ground), 陡下滑/圆拉平/浅下滑阶段(8/9/10)/1(Vwind_ground), 拉平/接地/滑跑刹车阶段(12/13/14)/4(Vwind_ground)
  MATLAB Function/1(gamma_cmd) -> 拉平/接地/滑跑刹车阶段(12/13/14)/2(gamma_cmd), 陡下滑/圆拉平/浅下滑阶段(8/9/10)/8(gamma_cmd), 进场/轨迹捕获阶段(6/7/8)/7(gamma_cmd)
  phi_eular/1 -> 陡下滑/圆拉平/浅下滑阶段(8/9/10)/6(phi_eular), 进场/轨迹捕获阶段(6/7/8)/5(phi_eular)
  Vg/1 -> MATLAB Function/4(Vg)
  进场/轨迹捕获阶段(6/7/8)/1(Cmd_Bus) -> Merge/1
  Compare To Constant1/1 -> AND/1
  拉平/接地/滑跑刹车阶段(12/13/14)/1(Cmd_Bus) -> Merge/3
  Compare To Constant/1 -> 进场/轨迹捕获阶段(6/7/8)/Enable
  Compare To Constant3/1 -> 拉平/接地/滑跑刹车阶段(12/13/14)/Enable
  Va_safe/1 -> 进场/轨迹捕获阶段(6/7/8)/2(Va_safe), 拉平/接地/滑跑刹车阶段(12/13/14)/5(Va_safe), 陡下滑/圆拉平/浅下滑阶段(8/9/10)/2(Va_safe)

== system takeoffANDlandingV5_23b/controller1/1_Pitch_Ctrl ==
  note: 起飞阶段：
      | 1.地面滑跑
      | 2.抬轮
      | 3.离地：
      | 4.爬升
      | 5.巡航
      | 降落阶段：
      | 6.进场飞行
      | 7.偏航轨迹捕获
      | 8.俯仰轨迹捕获
      | 9.陡下滑
      | 10.圆拉平
      | 11.浅下滑
      | 12.拉平
      | 13.接地
      | 14.地面滑跑
  Flight_Phase : Inport
  nz_cmd : Inport  Port=2
  theta_cmd : Inport  Port=3
  nz : Inport  Port=4
  theta : Inport  Port=5
  q : Inport  Port=6
  H_cmd : Inport  Port=7
  gamma : Inport  Port=8
  234俯仰角控制 : Subsystem
  5678三回路控制 : Subsystem
  910111213_着陆俯仰控制 : Subsystem
  Clock_blend : Clock
  Compare To Constant : simulink/Logic and Bit Operations/Compare To Constant  relop=>=  const=2  OutDataTypeStr=boolean
  Compare To Constant1 : simulink/Logic and Bit Operations/Compare To Constant  relop===  const=6  OutDataTypeStr=boolean
  Compare To Constant2 : simulink/Logic and Bit Operations/Compare To Constant  relop=<=  const=5  OutDataTypeStr=boolean
  Compare To Constant3 : simulink/Logic and Bit Operations/Compare To Constant  relop=>=  const=9  OutDataTypeStr=boolean
  Compare To Constant4 : simulink/Logic and Bit Operations/Compare To Constant  relop===  const=7  OutDataTypeStr=boolean
  Compare To Constant5 : simulink/Logic and Bit Operations/Compare To Constant  relop===  const=5  OutDataTypeStr=boolean
  Compare To Constant6 : simulink/Logic and Bit Operations/Compare To Constant  relop===  const=6  OutDataTypeStr=boolean
  Compare To Constant7 : simulink/Logic and Bit Operations/Compare To Constant  relop===  const=7  OutDataTypeStr=boolean
  Compare To Constant8 : simulink/Logic and Bit Operations/Compare To Constant  relop=<=  const=13  OutDataTypeStr=boolean
  Compare To Constant9 : simulink/Logic and Bit Operations/Compare To Constant  relop===  const=8  OutDataTypeStr=boolean
  Constant : Constant  Value=0
  Gain3 : Gain  Gain=HD
  Gain4 : Gain  Gain=HD
  Logical Operator : Logic  AllPortsSameDT=off  OutDataTypeStr=boolean
  Logical Operator1 : Logic  AllPortsSameDT=off  OutDataTypeStr=boolean
  Logical Operator2 : Logic  Operator=NOT  AllPortsSameDT=off  OutDataTypeStr=boolean
  Logical Operator3 : Logic  Operator=OR  Inputs=3  AllPortsSameDT=off  OutDataTypeStr=boolean
  Logical Operator4 : Logic  Operator=OR  Inputs=3  AllPortsSameDT=off  OutDataTypeStr=boolean
  Pitch45Blend : MATLAB Function  TreatAsAtomicUnit=on  SystemSampleTime=0.001
  Saturation : Saturate  UpperLimit=25  LowerLimit=-25
  Scope1 : Scope
  Switch : Switch  Criteria=u2 > Threshold  SaturateOnIntegerOverflow=off  InputSameDT=off
  Switch1 : Switch  Criteria=u2 > Threshold  SaturateOnIntegerOverflow=off  InputSameDT=off
  Switch2 : Switch  Criteria=u2 > Threshold  SaturateOnIntegerOverflow=off  InputSameDT=off
  T_blend : Constant  Value=5
  de_cmd : Outport
  wires:
  Flight_Phase/1 -> Compare To Constant8/1, Compare To Constant3/1, Compare To Constant9/1, Compare To Constant1/1, Compare To Constant4/1, Compare To Constant5/1, Compare To Constant6/1, Compare To Constant7/1, Pitch45Blend/1(phase), Compare To Constant/1, Compare To Constant2/1
  Gain3/1 -> Saturation/1
  theta_cmd/1 -> 234俯仰角控制/1(theta_cmd)
  theta/1 -> 234俯仰角控制/2(theta)
  nz_cmd/1 -> 5678三回路控制/1(nz_cmd)
  nz/1 -> 5678三回路控制/2(nz)
  q/1 -> 234俯仰角控制/3(q), 5678三回路控制/3(q)
  Logical Operator2/1 -> 5678三回路控制/4(复位)
  5678三回路控制/1(de_nz_rad) -> Gain4/1, Pitch45Blend/3(de_ny_rad)
  Compare To Constant1/1 -> Logical Operator3/2
  Compare To Constant4/1 -> Logical Operator3/1
  Logical Operator3/1 -> Switch/2
  [Vg] -> 910111213_着陆俯仰控制/1(Vg)
  H_cmd/1 -> 910111213_着陆俯仰控制/3(h_cmd)
  gamma/1 -> 910111213_着陆俯仰控制/2(gamma)
  Compare To Constant6/1 -> Logical Operator4/2
  Compare To Constant7/1 -> Logical Operator4/1
  Logical Operator4/1 -> Logical Operator2/1
  Compare To Constant5/1 -> Logical Operator4/3
  Gain4/1 -> Switch/1
  Compare To Constant/1 -> Logical Operator/1
  Compare To Constant2/1 -> Logical Operator/2
  Logical Operator/1 -> Switch1/2
  234俯仰角控制/1(de_theta_rad) -> Pitch45Blend/2(de_theta_rad)
  Clock_blend/1 -> Pitch45Blend/4(t)
  T_blend/1 -> Pitch45Blend/5(T_blend)
  Pitch45Blend/1(de_cmd_rad) -> Gain3/1
  Saturation/1 -> Switch1/1
  Pitch45Blend/2(lambda) -> Scope1/1
  Switch/1 -> Switch1/3
  Switch1/1 -> de_cmd/1
  Switch2/1 -> Switch/3
  Logical Operator1/1 -> Switch2/2
  Compare To Constant3/1 -> Logical Operator1/1
  Compare To Constant8/1 -> Logical Operator1/2
  910111213_着陆俯仰控制/1(de(D)) -> Switch2/1
  Constant/1 -> Switch2/3
  Compare To Constant9/1 -> Logical Operator3/3

== system takeoffANDlandingV5_23b/controller1/2_Yaw_Ctrl ==
  Flight_Phase : Inport
  Y : Inport  Port=2
  psi : Inport  Port=3
  r : Inport  Port=4
  psi_cmd : Inport  Port=5
  23456789101112段控制 : Subsystem
  Compare To Constant : simulink/Logic and Bit Operations/Compare To Constant  relop=>=  const=2  OutDataTypeStr=boolean
  Compare To Constant1 : simulink/Logic and Bit Operations/Compare To Constant  relop=<=  const=13  OutDataTypeStr=boolean
  Compare To Constant2 : simulink/Logic and Bit Operations/Compare To Constant  relop===  const=1  OutDataTypeStr=boolean
  Compare To Constant4 : simulink/Logic and Bit Operations/Compare To Constant  relop===  const=14  OutDataTypeStr=boolean
  Constant : Constant  Value=0
  Constant1 : Constant  Value=0
  Constant2 : Constant  Value=0
  Gain : Gain  Gain=HD
  Gain1 : Gain  Gain=HD
  Gain2 : Gain  Gain=-0.2
  Gain3 : Gain  Gain=-0.85
  K_z : Constant  Value=0.08
  Logical Operator : Logic  AllPortsSameDT=off  OutDataTypeStr=boolean
  Logical Operator1 : Logic  Operator=OR  AllPortsSameDT=off  OutDataTypeStr=boolean
  Product : Product
  Saturation : Saturate  UpperLimit=25  LowerLimit=-25
  Saturation1 : Saturate  UpperLimit=25  LowerLimit=-25
  Scope1 : Scope
  Sum : Sum  Inputs=|+-
  Sum1 : Sum  Inputs=|++
  Sum3 : Sum  Inputs=|++
  Switch : Switch  Criteria=u2 > Threshold  SaturateOnIntegerOverflow=off  InputSameDT=off
  Switch1 : Switch  Criteria=u2 > Threshold  SaturateOnIntegerOverflow=off  InputSameDT=off
  dr_cmd : Outport
  delta_s_cmd : Outport  Port=2
  wires:
  Gain/1 -> Saturation/1
  Saturation/1 -> dr_cmd/1
  Saturation1/1 -> delta_s_cmd/1
  Gain1/1 -> Saturation1/1
  Compare To Constant/1 -> Logical Operator/1
  Compare To Constant1/1 -> Logical Operator/2
  Logical Operator/1 -> Switch/2
  Compare To Constant2/1 -> Logical Operator1/1
  Logical Operator1/1 -> Switch1/2
  Constant/1 -> Switch1/3
  Flight_Phase/1 -> Compare To Constant/1, Compare To Constant1/1, Compare To Constant2/1, Compare To Constant4/1
  Constant1/1 -> Switch/3
  Switch1/1 -> Gain1/1
  Switch/1 -> Gain/1
  23456789101112段控制/1(dr_cmd) -> Switch/1
  Y/1 -> Sum/2, Scope1/1, 23456789101112段控制/1(Y)
  psi/1 -> Gain3/1, 23456789101112段控制/2(psi)
  r/1 -> Gain2/1, 23456789101112段控制/3(r)
  Gain3/1 -> Sum1/2
  Sum1/1 -> Sum3/1
  Gain2/1 -> Sum3/2
  Constant2/1 -> Sum/1
  Product/1 -> Sum1/1
  Sum/1 -> Product/2
  K_z/1 -> Product/1
  Sum3/1 -> Switch1/1
  Compare To Constant4/1 -> Logical Operator1/2
  psi_cmd/1 -> 23456789101112段控制/4(psi_cmd)

== system takeoffANDlandingV5_23b/controller1/3_Roll_Ctrl ==
  phi_cmd : Inport
  phi : Inport  Port=2
  p : Inport  Port=3
  Gain : Gain  Gain=180/pi
  Gain1 : Gain
  Gain2 : Gain  Gain=5
  Gain3 : Gain  Gain=0.1
  Gain4 : Gain  Gain=-1
  Integrator : Integrator
  Saturation : Saturate  UpperLimit=25  LowerLimit=-25
  Saturation1 : Saturate  UpperLimit=0.52  LowerLimit=-0.52
  Sum : Sum  Inputs=|+-
  Sum1 : Sum  Inputs=|++
  Sum2 : Sum  Inputs=|+-
  da_cmd : Outport
  wires:
  Gain/1 -> Saturation/1
  Saturation/1 -> Gain4/1
  phi_cmd/1 -> Sum/1
  phi/1 -> Sum/2
  Sum/1 -> Saturation1/1
  Gain3/1 -> Integrator/1
  Integrator/1 -> Sum1/2
  Gain2/1 -> Sum1/1
  Sum1/1 -> Sum2/1
  p/1 -> Sum2/2
  Sum2/1 -> Gain1/1
  Saturation1/1 -> Gain2/1, Gain3/1
  Gain1/1 -> Gain/1
  Gain4/1 -> da_cmd/1

== system takeoffANDlandingV5_23b/controller1/4_Power&V_Ctrl ==
  Flight_Phase : Inport
  throttle_cmd : Inport  Port=2
  V_cmd : Inport  Port=3
  V : Inport  Port=4
  brake_cmd : Inport  Port=5
  Clock_blend : Clock
  Compare To Constant1 : simulink/Logic and Bit Operations/Compare To Constant  relop=>=  const=1  OutDataTypeStr=boolean
  Compare To Constant2 : simulink/Logic and Bit Operations/Compare To Constant  relop=<=  const=5  OutDataTypeStr=boolean
  Compare To Constant3 : simulink/Logic and Bit Operations/Compare To Constant  relop=>=  const=6  OutDataTypeStr=boolean
  Compare To Constant5 : simulink/Logic and Bit Operations/Compare To Constant  relop=<=  const=13  OutDataTypeStr=boolean
  Constant : Constant  Value=5
  Constant3 : Constant  Value=0
  Delay1 : Delay  DelayLength=1
  Gain2 : Gain  Gain=0.1
  Gain3 : Gain  Gain=0.08
  Logical Operator : Logic  AllPortsSameDT=off  OutDataTypeStr=boolean
  Logical Operator1 : Logic  AllPortsSameDT=off  OutDataTypeStr=boolean
  MATLAB Function1 : MATLAB Function  TreatAsAtomicUnit=on
  MATLAB Function2 : MATLAB Function  TreatAsAtomicUnit=on
  Saturation1 : Saturate  UpperLimit=1  LowerLimit=0
  Saturation2 : Saturate  UpperLimit=1  LowerLimit=0
  Saturation3 : Saturate  UpperLimit=0.55  LowerLimit=-0.45
  Scope : Scope
  Sum4 : Sum  Inputs=|+-
  Sum5 : Sum  Inputs=|++
  Sum6 : Sum  Inputs=|+-
  Switch1 : Switch  Criteria=u2 > Threshold  SaturateOnIntegerOverflow=off  InputSameDT=off
  Switch2 : Switch  Criteria=u2 > Threshold  SaturateOnIntegerOverflow=off  InputSameDT=off
  平衡油门 : Constant  Value=0.3
  throttle : Outport
  u_brake_cmd : Outport  Port=2
  wires:
  Saturation1/1 -> u_brake_cmd/1
  brake_cmd/1 -> Saturation1/1
  Compare To Constant1/1 -> Logical Operator/1
  Compare To Constant2/1 -> Logical Operator/2
  Flight_Phase/1 -> MATLAB Function1/1(phase), Compare To Constant3/1, Compare To Constant5/1, Compare To Constant2/1, Compare To Constant1/1
  平衡油门/1 -> Sum5/2
  V/1 -> Sum6/2
  Sum6/1 -> Gain2/1
  Gain2/1 -> Sum4/1
  V_cmd/1 -> Sum6/1
  Sum4/1 -> Saturation3/1
  [vg_xyz] -> MATLAB Function2/1(Vel_g)
  Saturation3/1 -> Sum5/1
  Delay1/1 -> Gain3/1
  Sum5/1 -> MATLAB Function1/3(throttle_speed), Switch1/1
  MATLAB Function2/1(dv_err) -> Delay1/1
  Gain3/1 -> Sum4/2
  [a_xyz] -> MATLAB Function2/2(axyz)
  MATLAB Function1/1(throttle_out) -> Saturation2/1
  Clock_blend/1 -> MATLAB Function1/4(t)
  Constant/1 -> MATLAB Function1/5(T_blend)
  throttle_cmd/1 -> MATLAB Function1/2(throttle_direct)
  MATLAB Function1/2(lambda) -> Scope/1
  Logical Operator/1 -> Switch2/2
  Saturation2/1 -> Switch2/1
  Switch1/1 -> Switch2/3
  Logical Operator1/1 -> Switch1/2
  Compare To Constant3/1 -> Logical Operator1/1
  Compare To Constant5/1 -> Logical Operator1/2
  Constant3/1 -> Switch1/3
  Switch2/1 -> throttle/1

== system takeoffANDlandingV5_23b/controller1/刹车 ==
  u_brake_cmd : Inport
  Gain : Gain  Gain=1/0.1
  Integrator : Integrator  LimitOutput=on  UpperSaturationLimit=1  LowerSaturationLimit=0
  Sum : Sum  Inputs=|+-
  限制舵面角速度 : Saturate  UpperLimit=5  LowerLimit=-5
  u_brake : Outport
  wires:
  u_brake_cmd/1 -> Sum/1
  Sum/1 -> Gain/1
  Gain/1 -> 限制舵面角速度/1
  限制舵面角速度/1 -> Integrator/1
  Integrator/1 -> Sum/2, u_brake/1

== system takeoffANDlandingV5_23b/controller1/前轮 ==
  delta_s_cmd : Inport
  Gain : Gain  Gain=1/0.08
  Integrator : Integrator  LimitOutput=on  UpperSaturationLimit=25  LowerSaturationLimit=-25
  Sum : Sum  Inputs=|+-
  限制偏转速度 : Saturate  UpperLimit=120  LowerLimit=-120
  delta_s : Outport
  wires:
  delta_s_cmd/1 -> Sum/1
  Sum/1 -> Gain/1
  Gain/1 -> 限制偏转速度/1
  限制偏转速度/1 -> Integrator/1
  Integrator/1 -> Sum/2, delta_s/1

== system takeoffANDlandingV5_23b/controller1/副翼 ==
  da_cmd : Inport
  Gain : Gain  Gain=1/0.05
  Integrator : Integrator  LimitOutput=on  UpperSaturationLimit=25  LowerSaturationLimit=-25
  Sum : Sum  Inputs=|+-
  限制舵面角速度 : Saturate  UpperLimit=120  LowerLimit=-120
  da : Outport
  wires:
  da_cmd/1 -> Sum/1
  Sum/1 -> Gain/1
  Gain/1 -> 限制舵面角速度/1
  限制舵面角速度/1 -> Integrator/1
  Integrator/1 -> Sum/2, da/1

== system takeoffANDlandingV5_23b/controller1/升降舵 ==
  de_cmd : Inport
  Gain : Gain  Gain=1/0.08
  Integrator : Integrator  LimitOutput=on  UpperSaturationLimit=25  LowerSaturationLimit=-25
  Sum : Sum  Inputs=|+-
  限制舵面角速度 : Saturate  UpperLimit=50  LowerLimit=-50
  de : Outport
  wires:
  de_cmd/1 -> Sum/1
  Sum/1 -> Gain/1
  Gain/1 -> 限制舵面角速度/1
  限制舵面角速度/1 -> Integrator/1
  Integrator/1 -> Sum/2, de/1

== system takeoffANDlandingV5_23b/controller1/方向舵 ==
  dr_cmd : Inport
  Gain : Gain  Gain=1/0.05
  Integrator : Integrator  LimitOutput=on  UpperSaturationLimit=25  LowerSaturationLimit=-25
  Sum : Sum  Inputs=|+-
  限制舵面角速度 : Saturate  UpperLimit=100  LowerLimit=-100
  dr : Outport
  wires:
  Integrator/1 -> dr/1, Sum/2
  限制舵面角速度/1 -> Integrator/1
  Gain/1 -> 限制舵面角速度/1
  Sum/1 -> Gain/1
  dr_cmd/1 -> Sum/1
